simulink model "aero_model"  (R2024b)
settings: Solver=VariableStepAuto  StartTime=0.0  StopTime=10.0  RelTol=1e-3
settings Model: Creator=luis-albertosantiago  LastModifiedBy=luis-albertosantiago

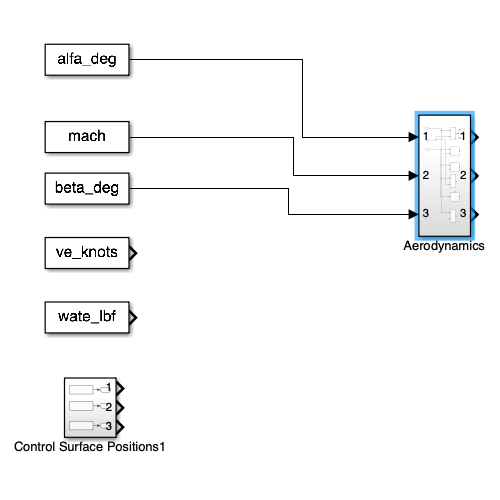
[thumbnail: Simulink's stored preview of the top-level diagram]
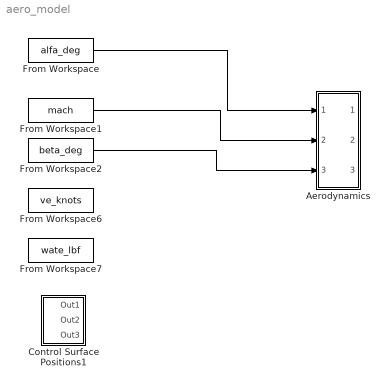
== system aero_model ==
  Aerodynamics : Subsystem
  Control Surface Positions1 : Subsystem
  From Workspace : FromWorkspace  VariableName=alfa_deg
  From Workspace1 : FromWorkspace  VariableName=mach
  From Workspace2 : FromWorkspace  VariableName=beta_deg
  From Workspace6 : FromWorkspace  VariableName=ve_knots
  From Workspace7 : FromWorkspace  VariableName=wate_lbf
  wires:
  From Workspace/1 -> Aerodynamics/1(In1)
  From Workspace2/1 -> Aerodynamics/3(In2)
  From Workspace1/1 -> Aerodynamics/2(In3)

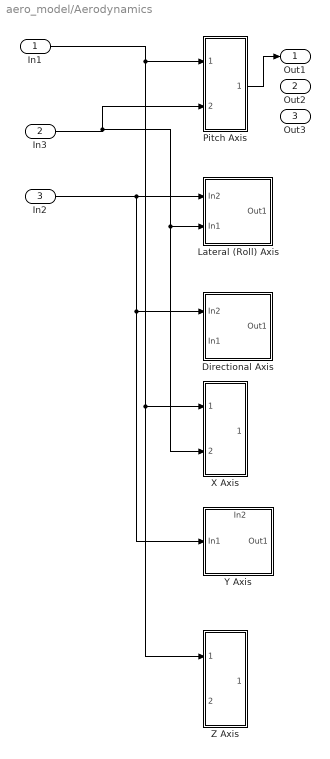
== system aero_model/Aerodynamics ==
  In1 : Inport
  In3 : Inport  Port=2
  In2 : Inport  Port=3
  Directional Axis : Subsystem
  Lateral (Roll) Axis : Subsystem
  Pitch Axis : Subsystem
  X Axis : Subsystem
  Y Axis : Subsystem
      settings: PortSchema="{\"entries\":[{\"content\":{\"sides\":[{\"content\":{\"connectorIds\":[\"In1\"]},\"type\":\"ConnectorPlacement.EquallySpacedRectSide\",\"uuid\":\"786a4368-23e1-4568-81be-c2b52f8c5df0\"},{\"content\":{\"connectorIds\":[\"Out1\"],\"side\":\"RIGHT\"},\"type\":\"ConnectorPlacement.EquallySpacedRectSide\",\"uuid\":\"e805c0ed-aaa8-4562-bd6b-82b12d681019\"},{\"content\":{\"connectorIds\":[\"In2\"],\"side\":\"TOP\"},\"type\":\"ConnectorPlacement.EquallySpacedRectSide\",\"uuid\":\"7d893d7b-794a-46a6-ab2d-de26fc0fccbd\"}]},\"type\":\"ConnectorPlacement.EquallySpacedConnector\",\"uuid\":\"e1b91ce4-f6cb-4e4b-9cc9-931b4bc15d2c\"}],\"packageUris\":[\"http://schema.mathworks.com/mf0/Connector/R2020b\"],\"version\":\"1.0\"}"
  Z Axis : Subsystem
  Out1 : Outport
  Out2 : Outport  Port=2
  Out3 : Outport  Port=3
  wires:
  In1/1 -> Z Axis/1(In3), X Axis/1(In5), Pitch Axis/1(In1)
  In2/1 -> Y Axis/1(In1), Directional Axis/1(In2), Lateral (Roll) Axis/1(In2)
  In3/1 -> Pitch Axis/2(In2), X Axis/2(In6), Lateral (Roll) Axis/2(In1)
  Pitch Axis/1(Out1) -> Out1/1
  ? -> Out2/1
  ? -> Out3/1

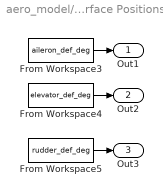
== system aero_model/Control Surface Positions1 ==
  From Workspace3 : FromWorkspace  VariableName=aileron_def_deg
  From Workspace4 : FromWorkspace  VariableName=elevator_def_deg
  From Workspace5 : FromWorkspace  VariableName=rudder_def_deg
  Out1 : Outport
  Out2 : Outport  Port=2
  Out3 : Outport  Port=3
  wires:
  From Workspace3/1 -> Out1/1
  From Workspace5/1 -> Out3/1
  From Workspace4/1 -> Out2/1

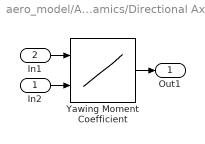
== system aero_model/Aerodynamics/Directional Axis ==
  In2 : Inport
  In1 : Inport  Port=2
  Yawing Moment Coefficient : Lookup_n-D  BreakpointsForDimension1=[1:3]  BreakpointsForDimension2=[1:3]  InternalRulePriority=Speed  RndMeth=Simplest
      settings: InputPortMap=u0,u1
  Out1 : Outport
  wires:
  In2/1 -> Yawing Moment Coefficient/2
  Yawing Moment Coefficient/1 -> Out1/1
  In1/1 -> Yawing Moment Coefficient/1

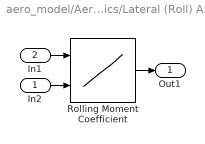
== system aero_model/Aerodynamics/Lateral (Roll) Axis ==
  In2 : Inport
  In1 : Inport  Port=2
  Rolling Moment Coefficient : Lookup_n-D  BreakpointsForDimension1=[1:3]  BreakpointsForDimension2=[1:3]  InternalRulePriority=Speed  RndMeth=Simplest
      settings: InputPortMap=u0,u1
  Out1 : Outport
  wires:
  Rolling Moment Coefficient/1 -> Out1/1
  In2/1 -> Rolling Moment Coefficient/2
  In1/1 -> Rolling Moment Coefficient/1

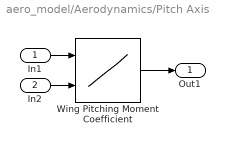
== system aero_model/Aerodynamics/Pitch Axis ==
  In1 : Inport
  In2 : Inport  Port=2
  Wing Pitching Moment Coefficient : Lookup_n-D  BreakpointsForDimension1=[1:3]  BreakpointsForDimension2=[1:3]  InternalRulePriority=Speed  RndMeth=Simplest
      settings: InputPortMap=u0,u1
  Out1 : Outport
  wires:
  Wing Pitching Moment Coefficient/1 -> Out1/1
  In2/1 -> Wing Pitching Moment Coefficient/2
  In1/1 -> Wing Pitching Moment Coefficient/1

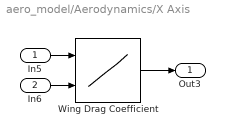
== system aero_model/Aerodynamics/X Axis ==
  In5 : Inport
  In6 : Inport  Port=2
  Wing Drag Coefficient : Lookup_n-D  BreakpointsForDimension1=[1:3]  BreakpointsForDimension2=[1:3]  InternalRulePriority=Speed  RndMeth=Simplest
      settings: InputPortMap=u0,u1
  Out3 : Outport
  wires:
  In6/1 -> Wing Drag Coefficient/2
  In5/1 -> Wing Drag Coefficient/1
  Wing Drag Coefficient/1 -> Out3/1

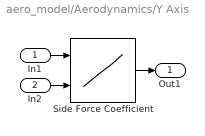
== system aero_model/Aerodynamics/Y Axis ==
  In1 : Inport
  In2 : Inport  Port=2
  Side Force Coefficient : Lookup_n-D  BreakpointsForDimension1=[1:3]  BreakpointsForDimension2=[1:3]  InternalRulePriority=Speed  RndMeth=Simplest
      settings: InputPortMap=u0,u1
  Out1 : Outport
  wires:
  In1/1 -> Side Force Coefficient/1
  In2/1 -> Side Force Coefficient/2
  Side Force Coefficient/1 -> Out1/1

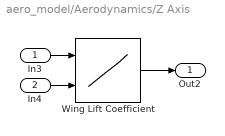
== system aero_model/Aerodynamics/Z Axis ==
  In3 : Inport
  In4 : Inport  Port=2
  Wing Lift Coefficient : Lookup_n-D  BreakpointsForDimension1=[1:3]  BreakpointsForDimension2=[1:3]  InternalRulePriority=Speed  RndMeth=Simplest
      settings: InputPortMap=u0,u1
  Out2 : Outport
  wires:
  Wing Lift Coefficient/1 -> Out2/1
  In3/1 -> Wing Lift Coefficient/1
  In4/1 -> Wing Lift Coefficient/2
